simulink model "task"  (R2015a)
settings: Solver=ode45  StartTime=0.0  StopTime=10.0  RelTol=1e-3
libraries: cstblocks x16
settings Model: Creator=saadc  LastModifiedBy=saadc

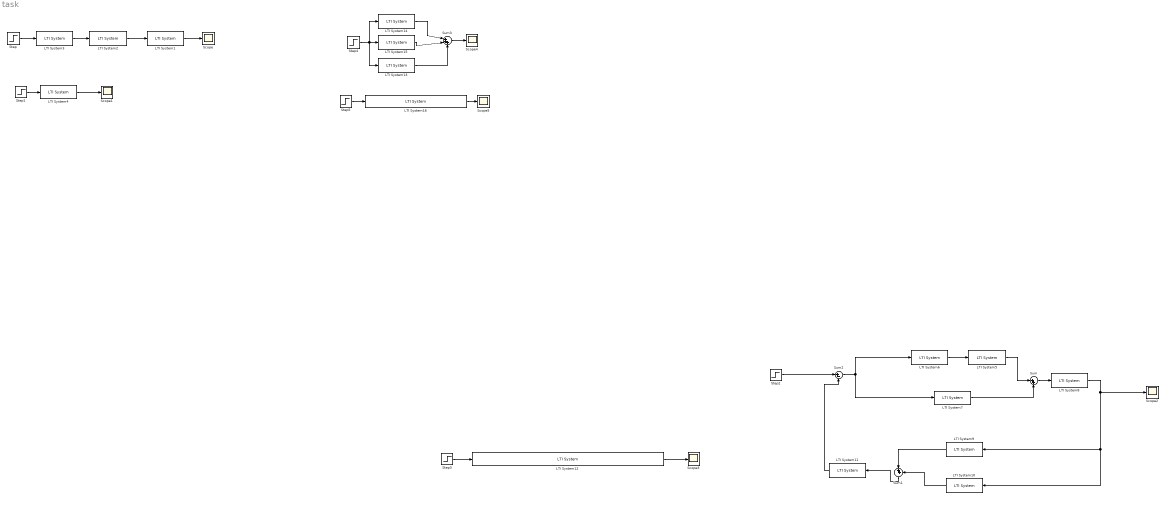
== system task ==
  LTI System{1,7..8,11,13} (5 alike) : cstblocks/LTI System  sys=tf([1 3],[1 5])  IC=[]
  LTI System{2,5,10,14} (4 alike) : cstblocks/LTI System  sys=tf(1,[1 4])  IC=[]
  LTI System12 : cstblocks/LTI System  sys=tf([1, 21, 183, 856, 2317, 3623, 3019, 1020],[1, 27, 291, 1634, 5144, 8974, 7916, 2765])  IC=[]
  LTI System{3,6,9,15} (4 alike) : cstblocks/LTI System  sys=tf(1,[1 1])  IC=[]
  LTI System16 : cstblocks/LTI System  sys=tf([1,10,34,37],[1, 10, 29 ,20])  IC=[]
  LTI System4 : cstblocks/LTI System  sys=tf([1,3],[1, 10, 29 ,20])  IC=[]
  Scope{,1..5} (6 alike) : Scope
      Scope2 settings: SaveName=ScopeData2
      Scope3 settings: SaveName=ScopeData3
      Scope4 settings: SaveName=ScopeData4
      Scope5 settings: SaveName=ScopeData5
  Step{,1..5} (6 alike) : Step  SampleTime=0
  Sum : Sum  Inputs=|++
  Sum1 : Sum  Inputs=|++
  Sum2 : Sum  Inputs=|+-
  Sum3 : Sum  Inputs=|+++
  wires:
  LTI System3/1 -> LTI System2/1
  LTI System2/1 -> LTI System1/1
  Step/1 -> LTI System3/1
  LTI System1/1 -> Scope/1
  LTI System6/1 -> LTI System5/1
  LTI System7/1 -> Sum/2
  LTI System5/1 -> Sum/1
  Sum/1 -> LTI System8/1
  LTI System9/1 -> Sum1/1
  LTI System10/1 -> Sum1/2
  Sum1/1 -> LTI System11/1
  LTI System8/1 -> Scope2/1, LTI System9/1, LTI System10/1
  LTI System11/1 -> Sum2/2
  Step2/1 -> Sum2/1
  Sum2/1 -> LTI System6/1, LTI System7/1
  Step1/1 -> LTI System4/1
  LTI System4/1 -> Scope1/1
  Step3/1 -> LTI System12/1
  LTI System12/1 -> Scope3/1
  Step4/1 -> LTI System13/1, LTI System14/1, LTI System15/1
  LTI System14/1 -> Sum3/1
  LTI System15/1 -> Sum3/2
  LTI System13/1 -> Sum3/3
  Sum3/1 -> Scope4/1
  Step5/1 -> LTI System16/1
  LTI System16/1 -> Scope5/1
